simulink model "ADU_Integration_R2014a_simulation"  (R2014a)
settings: Solver=FixedStepDiscrete  StartTime=285  StopTime=300  FixedStep=0.01  RelTol=1e-3
PostLoadFcn:
  | , if any(exist('dsrtsu_mdlpostloadfcn', 'file') == [2, 3, 6]), try dsrtsu_mdlpostloadfcn('Execute', bdroot); catch fprintf('Error in PostLoadFcn (dsrtsu_mdlpostloadfcn) for model "%s":\n %s\n', bdroot, lasterr); end, end,
InitFcn:
  | load 'data/chi2_dat';
  | load 'data/Line_struct';
  | load 'data/innerLNM_1';
  | load 'data/middleLNM_2';
  | load 'data/outerLNM_1';
  | load 'data/landmarks_patac_schimmel_ccw';
  | load 'data/patac_navi_array';
  | load 'data/sensor';
  | load 'data/map_struct';
  | addpath map_src
  | Integration_Parameter;
  | load 'TestData_001';
values from neighbouring files (symbols this model uses):
  TestData_001 =     [TestData_001.mat]
undefined symbols (not defined in the file or in its folder): chi2_dat, innerLNM_1, landmarks_patac_schimmel_ccw, middleLNM_2, outerLNM_1, patac_navi_array
libraries: simulink x36, rtican x1
(part 1 of 22)
settings Model: DSRTSU_INTERNAL_RTI_VER=460  DSRTSU_INTERNAL_RTI_TYPE=rti1401  DSRTSU_INTERNAL_RTIFLEXRAYCONFIG=10  DSRTSU_INTERNAL_RTIFPGA=50  Creator=si8cwy  LastModifiedBy=Administrator
settings DataIOCC: SignalLoggingSaveFormat=ModelDataLogs
settings OptimizationCC: BlockReduction=off  ConditionallyExecuteInputs=off  OptimizeBlockIOStorage=off  BufferReuse=off  GlobalBufferReuse=off  ExpressionFolding=off  ExpressionDepthLimit=2147483647  LocalBlockOutputs=off  RollThreshold=100
settings DebuggingCC: MergeDetectMultiDrivingBlocksExec=error  MultiTaskDSMMsg=warning  MultiTaskCondExecSysMsg=none  FrameProcessingCompatibilityMsg=error  StateNameClashWarn=warning
settings HardwareCC: ProdIntDivRoundTo=Zero  ProdEndianess=BigEndian  ProdHWDeviceType=Generic->Custom  TargetIntDivRoundTo=Zero  TargetEndianess=BigEndian  TargetHWDeviceType=Generic->Custom
settings RTWCC: SystemTargetFile=rti1401.tlc  MakeCommand=make_rti  TemplateMakefile=rti1401.tmf  Description=dSPACE DS1401 Hardware Platform
settings STFCustomTargetCC: ParMdlRefBuildCompliant=on  ConcurrentExecutionCompliant=off  GeneratePreprocessorConditionals=Use local settings  SystemTargetFile=rti1401.tlc
settings GRTTargetCC: CompOptLevelCompliant=off  ConcurrentExecutionCompliant=off  GeneratePreprocessorConditionals=Use local settings  CombineOutputUpdateFcns=off  MatFileLogging=off  CPPClassGenCompliant=off  GRTInterface=on  ExtModeMexFile=noextcomm

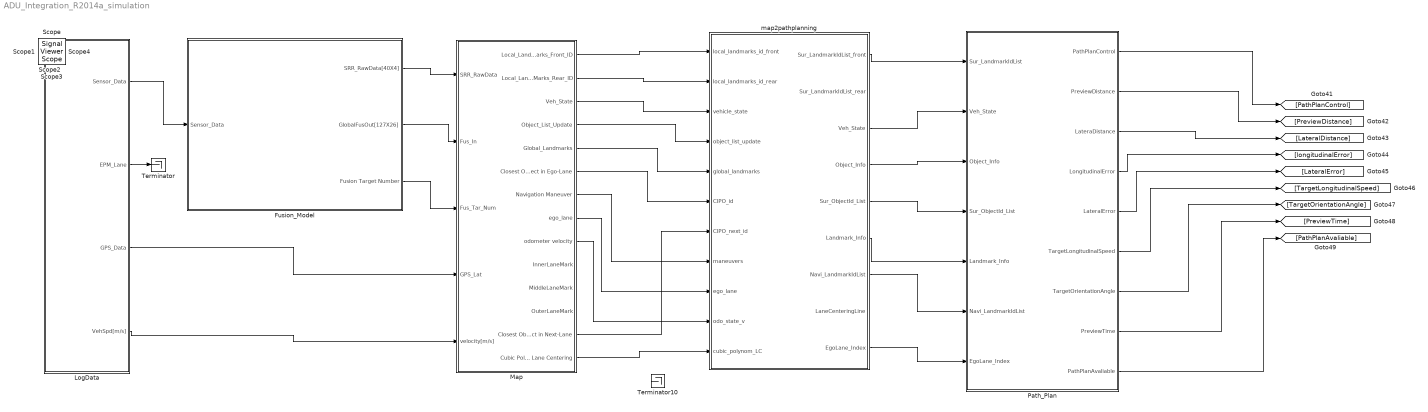
== system ADU_Integration_R2014a_simulation ==
  Fusion_Model : Subsystem
  LogData : Subsystem
  Map : Subsystem
  Path_Plan : Subsystem
  Terminator : Terminator
  Terminator10 : Terminator
  map2pathplanning : MATLAB Function  TreatAsAtomicUnit=on
      settings: PermitHierarchicalResolution=ParametersOnly
  Scope{,1..4} (5 alike) : SignalViewerScope  IOType=viewer  SampleTime=-1  ZoomMode=on
      Scope settings: TimeRange=auto  TickLabels=OneTimeTick  SaveToWorkspace=off  SaveName=ScopeData  YMin=-10  YMax=10  SampleInput=off
      Scope1 settings: TimeRange=auto  TickLabels=OneTimeTick  SaveToWorkspace=off  YMin=-10  YMax=10  SampleInput=off
      Scope2 settings: TimeRange=auto  TickLabels=OneTimeTick  SaveToWorkspace=off  SaveName=ScopeData2  YMin=-10  YMax=10  SampleInput=off
      Scope3 settings: TimeRange=auto  TickLabels=OneTimeTick  LimitDataPoints=on  SaveToWorkspace=off  SaveName=ScopeData3  YMin=-10  YMax=10  SampleInput=off
      Scope4 settings: TimeRange=auto  TickLabels=OneTimeTick  SaveToWorkspace=off  SaveName=ScopeData4  YMin=-10  YMax=10  SampleInput=off
  wires:
  LogData/1(Sensor_Data) -> Fusion_Model/1(Sensor_Data)
  LogData/2(EPM_Lane) -> Terminator/1
  Path_Plan/1(PathPlanControl) -> [PathPlanControl]
  Path_Plan/2(PreviewDistance) -> [PreviewDistance]
  Path_Plan/3(LateraDistance) -> [LateralDistance]
  Path_Plan/9(PathPlanAvaliable) -> [PathPlanAvaliable]
  Path_Plan/8(PreviewTime) -> [PreviewTime]
  Path_Plan/4(LongitudinalError) -> [longitudinalError]
  Path_Plan/5(LateralError) -> [LateralError]
  Path_Plan/7(TargetOrientationAngle) -> [TargetOrientationAngle]
  Path_Plan/6(TargetLongitudinalSpeed) -> [TargetLongitudinalSpeed]
  map2pathplanning/9(EgoLane_Index) -> Path_Plan/7(EgoLane_Index)
  map2pathplanning/7(Navi_LandmarkIdList) -> Path_Plan/6(Navi_LandmarkIdList)
  map2pathplanning/4(Object_Info) -> Path_Plan/3(Object_Info)
  map2pathplanning/1(Sur_LandmarkIdList_front) -> Path_Plan/1(Sur_LandmarkIdList)
  map2pathplanning/6(Landmark_Info) -> Path_Plan/5(Landmark_Info)
  Map/3(Veh_State) -> map2pathplanning/3(vehicle_state)
  Map/4(Object_List_Update) -> map2pathplanning/4(object_list_update)
  Map/5("Global_Landmarks ") -> map2pathplanning/5(global_landmarks)
  Map/6(Closest Object in Ego-Lane) -> map2pathplanning/6(CIPO_id)
  Map/7(Navigation Maneuver) -> map2pathplanning/8(maneuvers)
  Map/9(odometer velocity) -> map2pathplanning/10(odo_state_v)
  Fusion_Model/2(GlobalFusOut[127X26]) -> Map/2(Fus_In)
  Fusion_Model/1(SRR_RawData[40X4]) -> Map/1(SRR_RawData)
  LogData/3(GPS_Data) -> Map/4(GPS_Lat)
  LogData/4(VehSpd[m/s]) -> Map/5(velocity[m/s])
  Map/2(Local_LandMarks_Rear_ID) -> map2pathplanning/2(local_landmarks_id_rear)
  Fusion_Model/3(Fusion Target Number) -> Map/3(Fus_Tar_Num)
  Map/1(Local_LandMarks_Front_ID) -> map2pathplanning/1(local_landmarks_id_front)
  Map/8(ego_lane) -> map2pathplanning/9(ego_lane)
  map2pathplanning/3(Veh_State) -> Path_Plan/2(Veh_State)
  map2pathplanning/5(Sur_ObjectId_List) -> Path_Plan/4(Sur_ObjectId_List)
  Map/13(Closest Object in Next-Lane) -> map2pathplanning/7(CIPO_next_id)
  Map/14(Cubic Polynom for Lane Centering) -> map2pathplanning/11(cubic_polynom_LC)

== system ADU_Integration_R2014a_simulation/Fusion_Model ==
  note: SRR  Data
      | --------------------------------------------------------
      | |  1  |     2       |      3       |       4       |
      | --------------------------------------------------------
      | | ID | RangeX | RangeY | MoveInfo |
  note: Model Description:
      | This Model now don't take SRR Data to initial fusion tracker, the side fusion strategy will develop and update the model,
      | all output is based on vehicle coordinate, which original point located on the front middle of vehicle, the vehicle is 1.8m
      | wide and 5.2m long. Now the Move Info signal and Fus_State is unavialbe, The fusion output has two way, the 127x26
      | and 127 object is optional,the EPM Obstacle is used for ACC Strategy, not used for path plan and motion control.
  note: FusDataOut  Data
      | ------------------------------------------------------------------------------------------------------------------------------------------------------------------------------------------------------------------------------------------------------------------------------------------------------
      | |  1  |     2       |   3    |     4        |    5   |        6       |   7      |   8    |        9        |         10      |   11  |  12  |  13  |  14   | 15   |  16  |  17   |  18  |  19  |   20  |  21  |  22  |   23  |  24  |  25  |  26   |
      | -----------------------------------------------------------------------------------------------------------------------------------------------------------------------------------------------------------------------------------------------------------------------------------------------------
      | | ID | RangeX | VelX | RangeY | VelY | MoveInfo | Width | Type | Fus_State | Confidence| P11 | P12 | P13 | P14 | P21 | P22 | P23 | P24 | P31 | P32 | P33 | P34 | P41 | P42 | P43 | P44 |
  Sensor_Data : Inport
  DocBlock : simulink/Model-Wide Utilities/DocBlock  DocumentType=Text
      content=|
      | V1.0
      | 2016/11/1   |   First Release
      | V2.0
      | 2016/11/7   |   Changelog:
      | 1)  Output all SRR Raw Data, used for map;
      | 2)  Updating EPM dbc, new feature is avaliable;
      | 3)  Add Obstacle_State A/B/C for acc control;
      | 4)  Add FreeSpace and HPP signal for other use.
  Fusion_Block : Subsystem
  To Workspace : ToWorkspace  VariableName=FusOut  SampleTime=-1
  SRR_RawData[40X4] : Outport
  GlobalFusOut[127X26] : Outport  Port=2
  Fusion Target Number : Outport  Port=3
  wires:
  Fusion_Block/1(Fus_Data_Out) -> To Workspace/1, GlobalFusOut[127X26]/1
  Fusion_Block/3(SRR_RawData) -> SRR_RawData[40X4]/1
  Sensor_Data/1 -> Fusion_Block/1(Sensor_Data)
  Fusion_Block/2(fusion target number) -> Fusion Target Number/1

== system ADU_Integration_R2014a_simulation/LogData ==
  1-D Lookup Table2 : Lookup_n-D  NumberOfTableDimensions=1  BreakpointsForDimension1=TestData_001.X.Data  Table=TestData_001.Y(731).Data  RndMeth=Simplest  InputSameDT=on
  Bus Creator : BusCreator  Inputs=6
  Clock : Clock
  LF_SRR_Data : Subsystem
  LR_SRR_Data : Subsystem
  RF_SRR_Data : Subsystem
  RR_SRR_Data : Subsystem
  SER_M2S : Subsystem
  Sensor_ESR : Subsystem
  Vision_Target : Subsystem
  Sensor_Data : Outport
  EPM_Lane : Outport  Port=2
  GPS_Data : Outport  Port=3
  VehSpd[m/s] : Outport  Port=4
  tag scope: Clock=global
  wires:
  LF_SRR_Data/1(LF_SRR_Data[10x5]) -> Bus Creator/2  "LF_SRR_Data[10X5]"
  RF_SRR_Data/1(RF_SRR_Data[10x5]) -> Bus Creator/3  "RF_SRR_Data[10X5]"
  LR_SRR_Data/1(LR_SRR_Data[10x5]) -> Bus Creator/4  "LR_SRR_Data[10X5]"
  RR_SRR_Data/1(RR_SRR_Data[10x5]) -> Bus Creator/5  "RR_SRR_Data[10X5]"
  Vision_Target/1(Vision_Target[25x8]) -> Bus Creator/6  "Vision_Target[25X8]"
  Bus Creator/1 -> Sensor_Data/1  "Sensor_Veh_Data"
  Sensor_ESR/1(ESR_Data[64X4]) -> Bus Creator/1  "ESR_Data[64X4]"
  Vision_Target/2(EPM_Lane) -> EPM_Lane/1
  Clock/1 -> [Clock]
  SER_M2S/1(NET_Output) -> GPS_Data/1
  [Clock] -> 1-D Lookup Table2/1
  1-D Lookup Table2/1 -> VehSpd[m/s]/1

== system ADU_Integration_R2014a_simulation/Map ==
  SRR_RawData : Inport
  Fus_In : Inport  Port=2
  Fus_Tar_Num : Inport  Port=3
  GPS_Lat : Inport  Port=4
  velocity[m/s] : Inport  Port=5
  Bus Selector2 : BusSelector  OutputSignals=GPGLL.Y_Lat,GPGLL.Y_Long,GPHPR.Crouse_Range,GPGLL.Time[s]
  Constant : Constant  Value=chi2_dat
  Constant1 : Constant  Value=middleLNM_2  OutDataTypeStr=Bus: middleLine_struct
  Constant2 : Constant  Value=innerLNM_1  OutDataTypeStr=Bus: innerLine_struct
  Constant3 : Constant  Value=outerLNM_1  OutDataTypeStr=Bus: outerLine_struct
  Constant5 : Constant  Value=patac_navi_array  OutDataTypeStr=double
  Data Store Memory2 : DataStoreMemory  DataStoreName=chi2  ReadBeforeWriteMsg=warning  WriteAfterWriteMsg=warning  WriteAfterReadMsg=warning  InitialValue=zeros(1,1000)  ShowAdditionalParam=off  OutDataTypeStr=double
  Display : Display
  Map_Navigation : MATLAB Function  TreatAsAtomicUnit=on
      settings: PermitHierarchicalResolution=ParametersOnly
  Terminator{1..11} (11 alike) : Terminator
  landmarks_patac_schimmel_ccw : Constant  Value=landmarks_patac_schimmel_ccw  OutDataTypeStr=double
  Local_LandMarks_Front_ID : Outport
  Local_LandMarks_Rear_ID : Outport  Port=2
  Veh_State : Outport  Port=3
  Object_List_Update : Outport  Port=4
  "Global_Landmarks " : Outport  Port=5
  Closest Object in Ego-Lane : Outport  Port=6
  Navigation Maneuver : Outport  Port=7
  ego_lane : Outport  Port=8
  odometer velocity : Outport  Port=9
  InnerLaneMark : Outport  Port=10
  MiddleLaneMark : Outport  Port=11
  OuterLaneMark : Outport  Port=12
  Closest Object in Next-Lane : Outport  Port=13
  Cubic Polynom for Lane Centering : Outport  Port=14
  wires:
  velocity[m/s]/1 -> Map_Navigation/7(odo_motion_v)
  GPS_Lat/1 -> Bus Selector2/1
  Bus Selector2/1 -> Map_Navigation/8(rtk_gps_lat)  "<Y_Lat>"
  Bus Selector2/2 -> Map_Navigation/9(rtk_gps_lon)  "<Y_Long>"
  Bus Selector2/3 -> Map_Navigation/10(rtk_gps_yaw)  "<Crouse_Range>"
  Bus Selector2/4 -> Map_Navigation/11(rtk_gps_ts)  "<Time[s]>"
  SRR_RawData/1 -> Map_Navigation/12(sensor_data_raw)
  Fus_In/1 -> Map_Navigation/13(object_list)
  Constant/1 -> Map_Navigation/1(chi2_dat)
  Constant2/1 -> Map_Navigation/2(innerLine)
  Constant1/1 -> Map_Navigation/3(middleLine)
  Constant3/1 -> Map_Navigation/4(outerLine)
  landmarks_patac_schimmel_ccw/1 -> Map_Navigation/6(landmarks)
  Constant5/1 -> Map_Navigation/15(patac_navi)
  Fus_Tar_Num/1 -> Map_Navigation/14(object_num)
  Map_Navigation/3(object_list_update) -> Object_List_Update/1
  Map_Navigation/4(CIPO_id) -> Closest Object in Ego-Lane/1
  Map_Navigation/8(maneuvers) -> Navigation Maneuver/1
  Map_Navigation/25(step_out) -> Terminator4/1
  Map_Navigation/14(odo_state_v) -> odometer velocity/1
  Map_Navigation/1(global_landmarks) -> "Global_Landmarks "/1
  Map_Navigation/13(ego_location) -> ego_lane/1
  Map_Navigation/7(landmarks_in_proximity_id_in_rear) -> Local_LandMarks_Rear_ID/1
  Map_Navigation/6(landmarks_in_proximity_id_in_front) -> Local_LandMarks_Front_ID/1
  Map_Navigation/23(state_flag) -> Terminator2/1
  Map_Navigation/24(veh_ori_pos) -> Terminator1/1
  Map_Navigation/21(y_last) -> Terminator5/1
  Map_Navigation/22(v_last) -> Terminator3/1
  Map_Navigation/18(a_in_utm) -> Terminator8/1
  Map_Navigation/19(delta_t) -> Terminator7/1
  Map_Navigation/20(x_last) -> Terminator6/1
  Map_Navigation/15(t_in_utm) -> Terminator11/1
  Map_Navigation/16(x_in_utm) -> Terminator10/1
  Map_Navigation/17(y_in_utm) -> Terminator9/1
  Map_Navigation/9(innerLaneMark) -> InnerLaneMark/1
  Map_Navigation/10(middleLaneMark) -> MiddleLaneMark/1
  Map_Navigation/11(outerLaneMark) -> OuterLaneMark/1
  Map_Navigation/2(vehicle_state) -> Display/1, Veh_State/1
  Map_Navigation/5(CIPO_next_id) -> Closest Object in Next-Lane/1
  Map_Navigation/12(cubic_poly_coef) -> Cubic Polynom for Lane Centering/1

== system ADU_Integration_R2014a_simulation/Path_Plan ==
  note: Veh_State
      | |  1 |  2  |    3   |  4  |  5  |  6  |  7  | 8 |
      | -------------------------------------------------
      | | X  | Y  | Beta | Vx | Vy | Ax | Ay | V |
  note: FusDataOut  Data
      | ------------------------------------------------------------------------------------------------------------------------------------------------------------------------------------------------------------------------------------------------------
      | |  1  |     2       |   3    |     4        |    5   |        6       |   7      |   8    |        9        |         10      |   11  |  12  |  13  |  14   | 15   |  16  |  17   |  18  |  19  |   20  |  21  |  22  |   23  |  24  |  25  |  26   |
      | -------------------------------------------------------------------------------------------------------------------------------------------------------------------------------------------------------------------------------------------------------
      | | ID | RangeX | VelX | RangeY | VelY | MoveInfo | Width | Type | Fus_State | Confidence| P11 | P12 | P13 | P14 | P21 | P22 | P23 | P24 | P31 | P32 | P33 | P34 | P41 | P42 | P43 | P44 |
  note: Landmark_Info
      | |   1  |   2   |   3   |   4  |    5    |
      | ---------------------------------------- X 30
      | | X1  | Y1  |  X2  |  Y2 | Type |
  note: Sur_LandmarkIdList
      | |  1  |  2  |  3  |  4  |  5  |  6  |  7  |  8  |  9  |  10  |
      | --------------------------------------------------------------
      | | id  |
  note: Navi_LandmarkIdList
      | |  1  |  2  |      3      |    4   |
      | ----------------------------------
      | |  x  |  y  |  Range  |  OP  |
  note: Sur_ObjectId_List
      | |  1  |  2  |  3  |  4  |
      | -------------------------  1stLane   2ndLane  3rdLane
      | | id  |
  Sur_LandmarkIdList : Inport
  Veh_State : Inport  Port=2
  Object_Info : Inport  Port=3
  Sur_ObjectId_List : Inport  Port=4
  Landmark_Info : Inport  Port=5
  Navi_LandmarkIdList : Inport  Port=6
  EgoLane_Index : Inport  Port=7
  Constant : Constant
  CordTransfer : MATLAB Function  TreatAsAtomicUnit=on
      settings: PermitHierarchicalResolution=ParametersOnly
  CordTransfer1 : MATLAB Function  TreatAsAtomicUnit=on
      settings: PermitHierarchicalResolution=ParametersOnly
  Demux : Demux
  Demux1 : Demux
  Demux2 : Demux  Outputs=8
  InterSectionPathPlanningModule : Subsystem
  LaneChangePathPlanningModule1 : Subsystem
  PathArbModule : Subsystem
  SceneSelectionModule : Subsystem
  Terminator : Terminator
  Terminator1 : Terminator
  Terminator2 : Terminator
  Unit Delay : UnitDelay  InitialCondition=1  SampleTime=-1
  PathPlanControl : Outport
  PreviewDistance : Outport  Port=2
  LateraDistance : Outport  Port=3
  LongitudinalError : Outport  Port=4
  LateralError : Outport  Port=5
  TargetLongitudinalSpeed : Outport  Port=6
  TargetOrientationAngle : Outport  Port=7
  PreviewTime : Outport  Port=8
  PathPlanAvaliable : Outport  Port=9
  wires:
  Unit Delay/1 -> SceneSelectionModule/8(OperationFinishFlg)
  PathArbModule/6(PathTrigFinishFlg) -> Unit Delay/1
  LaneChangePathPlanningModule1/6(PathTrigFinishFlg) -> PathArbModule/12(PathTrigFinishFlgLC)
  InterSectionPathPlanningModule/6(PathTrigFinishFlg) -> PathArbModule/6(PathTrigFinishFlgInter)
  LaneChangePathPlanningModule1/5(PreViewTime) -> PathArbModule/11(PreviewTimeLC)
  LaneChangePathPlanningModule1/4(TargetThetalo) -> PathArbModule/10(TargetThetaLoLC)
  LaneChangePathPlanningModule1/3(PathPlanningSuccessFlg) -> PathArbModule/9(VePathPlan_e_LCPPSucFlg)
  LaneChangePathPlanningModule1/2(VsPathPlan_h_Motion) -> PathArbModule/8(VsPathPlan_h_LCMotion)
  LaneChangePathPlanningModule1/1(VsPathPlan_h_position) -> PathArbModule/7(VsPathPlan_h_LCposition)
  InterSectionPathPlanningModule/5(PreViewTime) -> PathArbModule/5(PreviewTimeInter)
  InterSectionPathPlanningModule/4(TargetThetalo) -> PathArbModule/4(TargetThetaLoInter)
  InterSectionPathPlanningModule/3(PathPlanningSuccessFlg) -> PathArbModule/3(VePathPlan_e_InterPPSucFlg)
  InterSectionPathPlanningModule/2(VsPathPlan_h_Motion) -> PathArbModule/2(VsPathPlan_h_InterSecMotion)
  InterSectionPathPlanningModule/1(VsPathPlan_h_position) -> PathArbModule/1(VsPathPlan_h_InterSecposition)
  PathArbModule/3(VePathPlan_b_InChargFlg) -> PathPlanControl/1
  PathArbModule/2(VsPathPlan_h_Motion) -> Demux1/1, CordTransfer1/3(VsPathPlan_h_MotionPGC)
  PathArbModule/1(VsPathPlan_h_position) -> Demux/1, CordTransfer1/2(VsPathPlan_h_positionPGC)
  PathArbModule/5(PreviewTime) -> PreviewTime/1
  PathArbModule/4(TargetThetaLo) -> TargetOrientationAngle/1, CordTransfer1/4(TargetThetaLoPGC)
  Demux1/1 -> TargetLongitudinalSpeed/1
  Demux/4 -> LateralError/1
  Demux/3 -> LongitudinalError/1
  Demux/2 -> LateraDistance/1
  Demux/1 -> PreviewDistance/1
  Constant/1 -> PathPlanAvaliable/1
  CordTransfer/6(Info_LoPGCd) -> LaneChangePathPlanningModule1/10(Info_Lo)
  CordTransfer/5(Info_LdPGCd) -> InterSectionPathPlanningModule/4(Info_Ld), LaneChangePathPlanningModule1/9(Info_Ld)
  CordTransfer/3(Info_FdPGCd) -> InterSectionPathPlanningModule/5(Info_Fd), LaneChangePathPlanningModule1/7(Info_Fd)
  Demux2/2 -> InterSectionPathPlanningModule/7(YposLoCur), LaneChangePathPlanningModule1/3(YposLoCur)
  Demux2/3 -> InterSectionPathPlanningModule/8(ThetaLoCur), LaneChangePathPlanningModule1/4(ThetaLoCur)
  CordTransfer/4(Info_FoPGCd) -> LaneChangePathPlanningModule1/8(Info_Fo)
  CordTransfer/1(Info_MePGCd) -> InterSectionPathPlanningModule/1(Info_Me), LaneChangePathPlanningModule1/1(Info_Me)
  Demux2/1 -> InterSectionPathPlanningModule/6(XposLoCur), LaneChangePathPlanningModule1/2(XposLoCur)
  CordTransfer/8(CurOpPGCd) -> InterSectionPathPlanningModule/3(VePathPlanning_e_CurOp), LaneChangePathPlanningModule1/6(VePathPlanning_e_CurOp), PathArbModule/13(VePathPlan_e_OutputSelection)
  Sur_LandmarkIdList/1 -> SceneSelectionModule/1(Sur_LandmarkIdList)
  Veh_State/1 -> Demux2/1, SceneSelectionModule/2(Veh_State)
  Navi_LandmarkIdList/1 -> SceneSelectionModule/6(Navi_LandmarkIdList)
  Landmark_Info/1 -> SceneSelectionModule/5(Landmark_Info)
  Sur_ObjectId_List/1 -> SceneSelectionModule/4(Sur_ObjectId_List)
  Object_Info/1 -> SceneSelectionModule/3(Object_Info)
  EgoLane_Index/1 -> SceneSelectionModule/7(EgoLane_Index)
  CordTransfer/2(RoadInfoPGCd) -> InterSectionPathPlanningModule/2(RoadInfo), LaneChangePathPlanningModule1/5(RoadInfo)
  CordTransfer/7(LongDisLimitPGCd) -> LaneChangePathPlanningModule1/11(LongDisLimit)
  SceneSelectionModule/1(Info_Me) -> CordTransfer/1(Info_MeGCd)
  SceneSelectionModule/2(Info_Fd) -> CordTransfer/2(Info_FdGCd)
  SceneSelectionModule/3(Info_Fo) -> CordTransfer/3(Info_FoGCd)
  SceneSelectionModule/5(Info_Lo) -> CordTransfer/5(Info_LoGCd)
  SceneSelectionModule/6(CurOp) -> CordTransfer/6(CurOpGCd)
  SceneSelectionModule/4(Info_Ld) -> CordTransfer/4(Info_LdGCd)
  SceneSelectionModule/7(LongDisLimit) -> CordTransfer/7(LongDisLimitGCd)
  SceneSelectionModule/8(RoadInfo) -> CordTransfer/8(RoadInfoGCd)
  CordTransfer/9(PGCdInfo) -> CordTransfer1/1(PGCdInfo)
  CordTransfer1/3(TargetThetaLo) -> Terminator2/1
  CordTransfer1/2(VsPathPlan_h_Motion) -> Terminator1/1
  CordTransfer1/1(VsPathPlan_h_position) -> Terminator/1

== system ADU_Integration_R2014a_simulation/Fusion_Model/Fusion_Block ==
  Sensor_Data : Inport
  Bus Selector : BusSelector  OutputSignals=Total_Targ_Num
  Display : Display
  Fus_Header_Gen : Subsystem
  Global_Fusion : Subsystem
  Side_Fusion : Subsystem
  Terminator : Terminator
  Fus_Data_Out : Outport
  fusion target number : Outport  Port=2
  SRR_RawData : Outport  Port=3
  wires:
  Side_Fusion/1(SideFus_Output[40X4]) -> Global_Fusion/1(From SideFusion)
  Global_Fusion/1(GlobalFusOut[127X26]) -> Fus_Data_Out/1
  Sensor_Data/1 -> Side_Fusion/1(From Sensor), Global_Fusion/2(From Sensor)
  Global_Fusion/2(Total_TargetNum) -> Display/1, Fus_Header_Gen/1(Target_Num)
  Side_Fusion/2(SideRadar_RawData[40X4]) -> SRR_RawData/1
  Fus_Header_Gen/1(Fus_Header) -> Bus Selector/1, Terminator/1
  Bus Selector/1 -> fusion target number/1  "<Total_Targ_Num>"

== system ADU_Integration_R2014a_simulation/LogData/LF_SRR_Data ==
  note: This part is used for ensure the sensor data is from once update
  1-D Lookup Table : Lookup_n-D  NumberOfTableDimensions=1  BreakpointsForDimension1=TestData_001.X.Data  Table=TestData_001.Y(51).Data  RndMeth=Simplest  InputSameDT=on
  Chart : Stateflow chart  TreatAsAtomicUnit=on
      settings: PermitHierarchicalResolution=ParametersOnly
  LFSRR_Data : Subsystem
  LF_SRR_Data[10x5] : Outport
  tag scope: LFSRRTime=global, LFSRRcal=global
  wires:
  LFSRR_Data/1(LFSRR[10X5]) -> Chart/2(DataInput)
  1-D Lookup Table/1 -> Chart/1(Trig), [LFSRRcal]
  Chart/1(DataOutput) -> LF_SRR_Data[10x5]/1
  [Clock] -> Chart/3(Time), 1-D Lookup Table/1
  Chart/2(Time_out) -> [LFSRRTime]

== system ADU_Integration_R2014a_simulation/LogData/LR_SRR_Data ==
  1-D Lookup Table : Lookup_n-D  NumberOfTableDimensions=1  BreakpointsForDimension1=TestData_001.X.Data  Table=TestData_001.Y(51*2).Data  RndMeth=Simplest  InputSameDT=on
  Chart : Stateflow chart  TreatAsAtomicUnit=on
      settings: PermitHierarchicalResolution=ParametersOnly
  LRSRR_Data : Subsystem  mask{StartNum=52}
  Rate Transition3 : RateTransition  Deterministic=off
  LR_SRR_Data[10x5] : Outport
  tag scope: LRSRRTime=global, LRSRRcal=global
  wires:
  Chart/1(DataOutput) -> Rate Transition3/1
  1-D Lookup Table/1 -> Chart/1(Trig), [LRSRRcal]
  Rate Transition3/1 -> LR_SRR_Data[10x5]/1
  [Clock] -> Chart/3(Time), 1-D Lookup Table/1
  LRSRR_Data/1(LRSRR[10X5]) -> Chart/2(DataInput)
  Chart/2(Time_out) -> [LRSRRTime]

== system ADU_Integration_R2014a_simulation/LogData/RF_SRR_Data ==
  1-D Lookup Table : Lookup_n-D  NumberOfTableDimensions=1  BreakpointsForDimension1=TestData_001.X.Data  Table=TestData_001.Y(153).Data  RndMeth=Simplest  InputSameDT=on
  Chart : Stateflow chart  TreatAsAtomicUnit=on
      settings: PermitHierarchicalResolution=ParametersOnly
  RFSRR_Data : Subsystem  mask{StartNum=103}
  RF_SRR_Data[10x5] : Outport
  tag scope: RFSRRTime=global, RFSRRcal=global
  wires:
  1-D Lookup Table/1 -> Chart/1(Trig), [RFSRRcal]
  Chart/1(DataOutput) -> RF_SRR_Data[10x5]/1
  [Clock] -> Chart/3(Time), 1-D Lookup Table/1
  RFSRR_Data/1(RFSRR[10X5]) -> Chart/2(DataInput)
  Chart/2(Time_out) -> [RFSRRTime]

== system ADU_Integration_R2014a_simulation/LogData/RR_SRR_Data ==
  1-D Lookup Table : Lookup_n-D  NumberOfTableDimensions=1  BreakpointsForDimension1=TestData_001.X.Data  Table=TestData_001.Y(51*4).Data  RndMeth=Simplest  InputSameDT=on
  Chart : Stateflow chart  TreatAsAtomicUnit=on
      settings: PermitHierarchicalResolution=ParametersOnly
  LRSRR_Data : Subsystem  mask{StartNum=154}
  RR_SRR_Data[10x5] : Outport
  tag scope: RRSRRTime=global, RRSRRcal=global
  wires:
  LRSRR_Data/1(RRSRR[10X5]) -> Chart/2(DataInput)
  [Clock] -> Chart/3(Time), 1-D Lookup Table/1
  1-D Lookup Table/1 -> Chart/1(Trig), [RRSRRcal]
  Chart/1(DataOutput) -> RR_SRR_Data[10x5]/1
  Chart/2(Time_out) -> [RRSRRTime]

== system ADU_Integration_R2014a_simulation/LogData/SER_M2S ==
  1-D Lookup Table1 : Lookup_n-D  NumberOfTableDimensions=1  BreakpointsForDimension1=TestData_001.X.Data  Table=TestData_001.Y(739).Data  RndMeth=Simplest  InputSameDT=on
  1-D Lookup Table2 : Lookup_n-D  NumberOfTableDimensions=1  BreakpointsForDimension1=TestData_001.X.Data  Table=TestData_001.Y(738).Data  RndMeth=Simplest  InputSameDT=on
  1-D Lookup Table3 : Lookup_n-D  NumberOfTableDimensions=1  BreakpointsForDimension1=TestData_001.X.Data  Table=TestData_001.Y(740).Data  RndMeth=Simplest  InputSameDT=on
  1-D Lookup Table4 : Lookup_n-D  NumberOfTableDimensions=1  BreakpointsForDimension1=TestData_001.X.Data  Table=TestData_001.Y(740).Data  RndMeth=Simplest  InputSameDT=on
  1-D Lookup Table5 : Lookup_n-D  NumberOfTableDimensions=1  BreakpointsForDimension1=TestData_001.X.Data  Table=TestData_001.Y(734).Data  RndMeth=Simplest  InputSameDT=on
  1-D Lookup Table6 : Lookup_n-D  NumberOfTableDimensions=1  BreakpointsForDimension1=TestData_001.X.Data  Table=TestData_001.Y(735).Data  RndMeth=Simplest  InputSameDT=on
  1-D Lookup Table7 : Lookup_n-D  NumberOfTableDimensions=1  BreakpointsForDimension1=TestData_001.X.Data  Table=TestData_001.Y(736).Data  RndMeth=Simplest  InputSameDT=on
  Bus Creator : BusCreator  Inputs=3
  Bus Creator1 : BusCreator  Inputs=4
  Bus Creator2 : BusCreator  Inputs=2
  NET_Output : Outport
  wires:
  1-D Lookup Table3/1 -> Bus Creator/3  "Time[s]"
  1-D Lookup Table2/1 -> Bus Creator/1  "Y_Lat"
  1-D Lookup Table1/1 -> Bus Creator/2  "Y_Long"
  Bus Creator2/1 -> NET_Output/1
  Bus Creator1/1 -> Bus Creator2/2  "GPHPR"
  1-D Lookup Table6/1 -> Bus Creator1/3  "Pitch_angle"
  1-D Lookup Table5/1 -> Bus Creator1/2  "Crouse_Range"
  Bus Creator/1 -> Bus Creator2/1  "GPGLL"
  1-D Lookup Table4/1 -> Bus Creator1/1  "Time"
  1-D Lookup Table7/1 -> Bus Creator1/4  "Roll_angle"
  [Clock] -> 1-D Lookup Table2/1, 1-D Lookup Table1/1, 1-D Lookup Table7/1, 1-D Lookup Table6/1, 1-D Lookup Table5/1, 1-D Lookup Table4/1, 1-D Lookup Table3/1
